simulink model "OPAMsimulink"  (R2024b)
settings: Solver=VariableStepAuto  StartTime=0.0  StopTime=2  RelTol=1e-3
InitFcn:
  | R1=5e6;
  | R2=R1;
  | R3=R1;
  | C1=100e-9;
  | C2=C1;

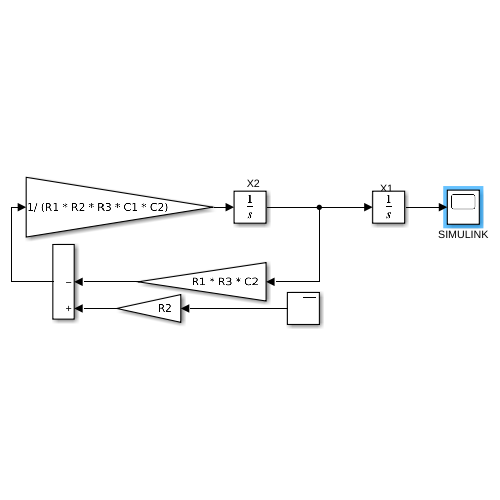
[thumbnail: Simulink's stored preview of the top-level diagram]
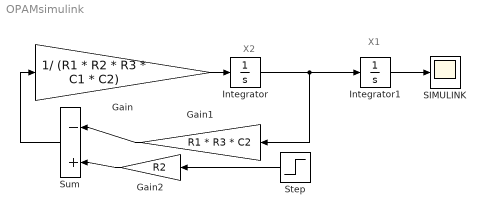
== system OPAMsimulink ==
  note: X2
  note: X1
  Gain : Gain  Gain=1/ (R1 * R2 * R3 * C1 * C2)
  Gain1 : Gain  Gain=R1 * R3 * C2
  Gain2 : Gain  Gain=R2
  Integrator : Integrator
  Integrator1 : Integrator
  SIMULINK : Scope
  Step : Step  Time=0  After=5  SampleTime=0
  Sum : Sum  Inputs=|-+
  wires:
  Integrator/1 -> Gain1/1, Integrator1/1
  Integrator1/1 -> SIMULINK/1
  Gain2/1 -> Sum/2
  Step/1 -> Gain2/1
  Gain1/1 -> Sum/1
  Sum/1 -> Gain/1
  Gain/1 -> Integrator/1
